simulink model "base_model"  (R2025b)
settings: Solver=VariableStepAuto  StartTime=0.0  StopTime=10.0  RelTol=1e-3
undefined symbols (not defined in the file or in its folder): myGain
settings Model: Creator=KoayXianCong  LastModifiedBy=KoayXianCong

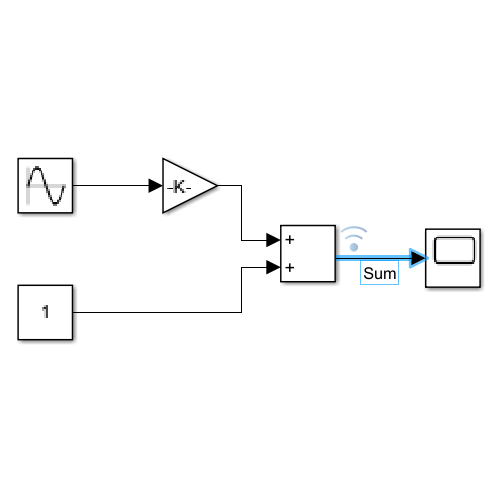
[thumbnail: Simulink's stored preview of the top-level diagram]
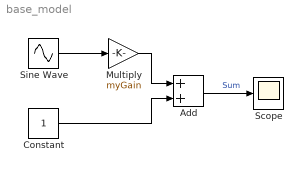
== system base_model ==
  Add : Sum
  Constant : Constant
  Multiply : Gain  Gain=myGain
  Scope : Scope
      settings: ActiveDisplayYMinimum=-1  ActiveDisplayYMaximum=1
  Sine Wave : Sin  SampleTime=0
  wires:
  Sine Wave/1 -> Multiply/1
  Multiply/1 -> Add/1
  Constant/1 -> Add/2
  Add/1 -> Scope/1  "Sum"
